simulink model "test_simulink"  (R2013a)
settings: Solver=FixedStepDiscrete  StartTime=0.0  StopTime=100.0  RelTol=1e-3
values from neighbouring files (symbols this model uses):
  at = 1e-4    (= 0.0001)    [simu_ini.m]
  buff_size = frame_len    [simu2_ini.m]    (also in simu_ini.m = 11025)
  detect_pow = 0.3    [simu_ini.m]
  Fs = 22050    [simu_ini.m]
  rt = 50e-3    (= 0.05)    [simu_ini.m]
  samp_range_search = 100    [simu_ini.m]
  thres = 0.4    [simu_ini.m]
  time_left = 2e-3    (= 0.002)    [simu_ini.m]
  time_right = 20e-3    (= 0.02)    [simu_ini.m]
undefined symbols (not defined in the file or in its folder): get
libraries: simulink x2, dspmlti4 x1, dspsrcs4 x1, dspnetwork x1, dspsnks4 x1
settings Model: Creator=leonardo  LastModifiedBy=leonardo

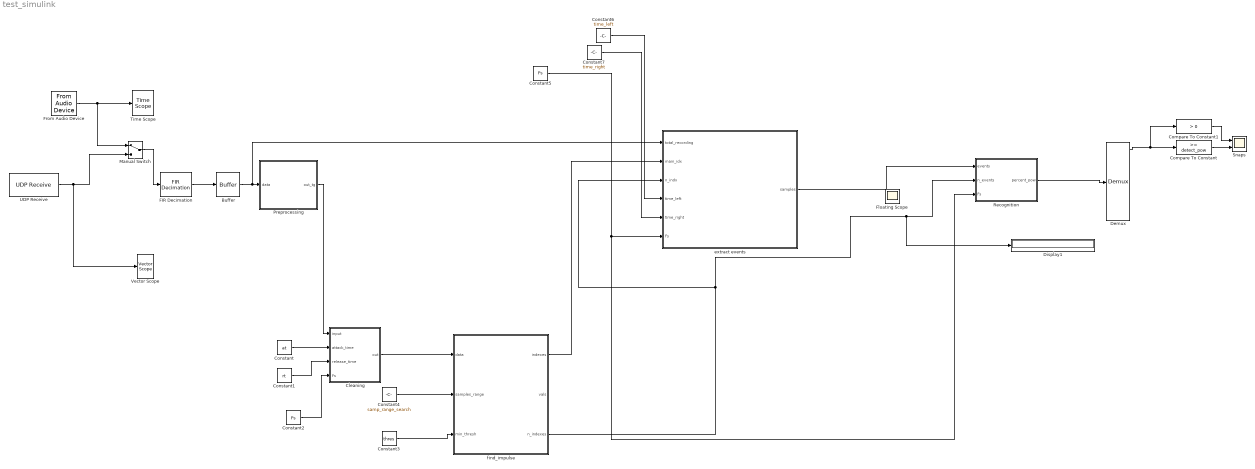
== system test_simulink ==
  Buffer : Buffer  N=buff_size  TreatMby1Signals=One channel
  Cleaning : MATLAB Function  TreatAsAtomicUnit=on
  Compare To Constant : simulink/Logic and Bit Operations/Compare To Constant  relop=>=  const=detect_pow  OutDataTypeStr=boolean
  Compare To Constant1 : simulink/Logic and Bit Operations/Compare To Constant  relop=>  const=0  OutDataTypeStr=boolean
  Constant : Constant  Value=at
  Constant1 : Constant  Value=rt
  Constant2 : Constant  Value=Fs
  Constant3 : Constant  Value=thres
  Constant4 : Constant  Value=samp_range_search
  Constant5 : Constant  Value=Fs
  Constant6 : Constant  Value=time_left
  Constant7 : Constant  Value=time_right
  Demux : Demux  Outputs=10
  Display1 : Display
  FIR Decimation : dspmlti4/FIR Decimation  h=fir1(35,0.4)  D=2  filtStruct=Direct form  framing=Enforce single-rate processing  inputOffset=0  outputBufInitCond=0  InputProcessing=Columns as channels (frame based)  firstCoeffDataTypeStr=Inherit: Same word length as input  firstCoeffLastDataTypeStr=Inherit: Same word length as input  firstCoeffMin=[]  firstCoeffMax=[]  outputDataTypeStr=Inherit: Same as accumulator  outputLastDataTypeStr=Inherit: Same as accumulator  outputMin=[]  outputMax=[]  roundingMode=Floor  overflowMode=off  FilterSource=Specify via dialog  FilterObject=Hm_firdecim
      settings: allowOverrides=off
  Floating Scope : Scope
      settings: Floating=on
  From Audio Device : dspsrcs4/From Audio Device  deviceName=Default  numChannels=1  sampleRate=44100  deviceDatatype=32-bit float  autoBufferSize=on  bufferSize=4096  queueDuration=1.0  frameSize=2048  outputDatatype=single
  Manual Switch : ManualSwitch
  Preprocessing : MATLAB Function  TreatAsAtomicUnit=on
  Recognition : MATLAB Function  TreatAsAtomicUnit=on
  Snaps : Scope  NumInputPorts=2
      settings: YMin=-5~-5  YMax=5~5
  Time Scope : TimeScope  DefaultConfigurationName=spbscopes.TimeScopeBlockCfg
      settings: CopyFcn=scopeextensions.ScopeBlock.callback(gcbh, 'onBlockCopy', gcbh);  DeleteFcn=scopeextensions.ScopeBlock.callback(gcbh, 'onBlockDelete');  PreSaveFcn=scopeextensions.ScopeBlock.callback(gcbh, 'onModelSave');  NameChangeFcn=scopeextensions.ScopeBlock.callback(gcbh, 'onBlockRename');  CloseFcn=scopeextensions.ScopeBlock.callback(gcbh, 'onBlockClose');  PreDeleteFcn=scopeextensions.ScopeBlock.callback(gcbh, 'onBlockPreDelete');
  UDP Receive : dspnetwork/UDP Receive  localURL='0.0.0.0'  localPort=9090  remoteURL='192.168.2.1'  remotePort=-1  recvBufferSize=2048  dims=255  signalDatatype=int16  isVarSize=on  showBlockingTime=off  blockingTime=0  sampletime=1
  Vector Scope : dspsnks4/Vector Scope  ScopeProperties=on  Domain=Time  HorizSpan=1  DisplayProperties=off  AxisGrid=on  Memory=on  FrameNumber=on  AxisLegend=off  AxisZoom=off  OpenScopeAtSimStart=on  OpenScopeImmediately=off  FigPos=get(0,'defaultfigureposition')  AxisProperties=off  XUnits=Hertz  XRange=[0...Fs/2]  InheritXIncr=on  XIncr=1  XLabel=Time  XLimit=Auto  XMin=0  XMax=1  XStart=0  YUnits=dB  YLabel=Amplitude  LineProperties=off  XAxisParamsVer=6.9
      settings: YMin=-10  YMax=10
  extract events : MATLAB Function  TreatAsAtomicUnit=on
  find_impulse : MATLAB Function  TreatAsAtomicUnit=on
  wires:
  Constant/1 -> Cleaning/2(attack_time)
  Constant1/1 -> Cleaning/3(release_time)
  Cleaning/1(out) -> find_impulse/1(data)
  Preprocessing/1(out_tg) -> Cleaning/1(input)
  Constant3/1 -> find_impulse/3(min_thresh)
  Constant4/1 -> find_impulse/2(samples_range)
  Constant6/1 -> extract events/4(time_left)
  Constant7/1 -> extract events/5(time_right)
  find_impulse/1(indexes) -> extract events/2(main_idx)
  Buffer/1 -> extract events/1(total_recording), Preprocessing/1(data)
  extract events/1(samples) -> Recognition/1(events)
  find_impulse/3(n_indexes) -> Display1/1, Recognition/2(n_events), extract events/3(n_indx)
  Recognition/1(percent_pow) -> Demux/1
  FIR Decimation/1 -> Buffer/1
  Constant2/1 -> Cleaning/4(Fs)
  Constant5/1 -> Recognition/3(Fs), extract events/6(Fs)
  Demux/1 -> Compare To Constant1/1, Compare To Constant/1
  Compare To Constant/1 -> Snaps/2
  Compare To Constant1/1 -> Snaps/1
  From Audio Device/1 -> Manual Switch/1, Time Scope/1
  Manual Switch/1 -> FIR Decimation/1
  UDP Receive/1 -> Vector Scope/1, Manual Switch/2

== matlab function test_simulink/Cleaning ==
  data: input input; out output; attack_time input; release_time input; Fs input
function out=xrms2(input,attack_time,release_time,Fs)

local_peak=abs(input(1));
len=length(input);
at = 1-exp(-2.2/(Fs*attack_time));
rt = 1-exp(-2.2/(Fs*release_time));
out=zeros(1,len);

out(1)=local_peak;

for i=2:len
    
    a=abs(input(i));
    
    if a > local_peak
        
        coeff = at;
        
    else
        
        coeff = rt;
    end
    
    local_peak = (1-coeff)*local_peak+coeff*a;
      
    out(i)=local_peak;

end

== matlab function test_simulink/Preprocessing ==
  data: data input; out_tg output
function out_tg =detect_energy_threshold(data)



out_tg=prep(data);



end

function y = prep(x)



x=x(:); 

L = length(x);

y = x(2:L-1).^2-x(1:L-2).*x(3:L);
y = [y(1); y; y(L-2)];

end

== matlab function test_simulink/find_impulse ==
  data: data input; indexes output; samples_range input; min_thresh input; vals output; n_indexes output
function [indexes,vals,n_indexes]=find_local_max(data,samples_range,min_thresh)

len = length(data);
indexes=zeros(1,len);
vals=zeros(1,len);
k=1;
% max_sample_range=500;
% idx_l=zeros(1,max_sample_range);
% idx_r=zeros(1,max_sample_range);


for i = samples_range+1 : len -samples_range -1
    
%     idx_l(1,1:samples_range) = i-1:-1:i-samples_range;
%     idx_r(1,1:samples_range)  = i+1:i+samples_range;
skip = 0;
    if data(i)<=min_thresh
        skip=1;
    else
         for j=i+1:1:i+samples_range
            a2 =  data(i)> data(j);
            if a2==0
                skip=1;
                break;
            end
         end
        if skip==0
            for j = i-1:-1:i-samples_range 
                a1 =  data(i)> data(j);
                if a1==0
                    skip=1;
                    break;
                end
            end
        end
       
    end
 
    if skip==0

        indexes(k)=i;
        vals(k)=data(i);
        k=k+1;
    end

end

n_indexes=k-1;
end

== matlab function test_simulink/extract events ==
  data: samples output; total_recording input; main_idx input; n_indx input; time_left input; time_right input; Fs input
function samples   = extract_events( total_recording,main_idx,n_indx,time_left,time_right,Fs)


max_idx=10;
% global Fs;
% n_indx=length(main_idx);
n_max_samples = ceil(50e-3*22050);%max_len*Fs;
 samples=zeros(max_idx,n_max_samples);
% sample_left=zeros(1,n_idx);
% sample_right=zeros(1,n_idx);
samp_len=zeros(max_idx,1);

if n_indx>max_idx
    fprintf('too much indexes');
    
end

if n_indx>=1

for i=1:n_indx
    
    sample_left = fix(main_idx(i)-time_left*Fs);
    sample_right = ceil(main_idx(i)+time_right*Fs);
    if sample_right>length(total_recording)
        sample_right=length(total_recording);
    end
    extract_len=sample_right-sample_left+1;
   
     samples(i,1:extract_len)=total_recording(sample_left:sample_right);
    
end

end


end

== matlab function test_simulink/Recognition ==
  data: events input; percent_pow output; n_events input; Fs input
function percent_pow = snap_recognition(events,n_events,Fs)


frq_sx=1500;
frq_dx=3000;

len_fft=512;


freq_step=Fs/(len_fft-1);
sx_bin=round(frq_sx/freq_step)+1;
dx_bin=round(frq_dx/freq_step)+1;
max_events=10;
percent_pow=zeros(1,max_events);
% fft_axe=0:freq_step:Fs;
if n_events>max_events
    error('too much events');
end

if n_events>=1

    for i=1:n_events

        ff = abs(fft(events(i,1:len_fft)).^2);
        tot_pow = sum(ff(1:len_fft/2));
        sel_pow = sum(ff(sx_bin:dx_bin));
        percent_pow(i)=sel_pow/tot_pow;
    end

end
